simulink model "project4"  (R2020b)
settings: Solver=VariableStepAuto  StartTime=0.0  StopTime=5  RelTol=1e-3
libraries: simulink x1, commutil2 x1
settings Model: Creator=derek  LastModifiedBy=hp

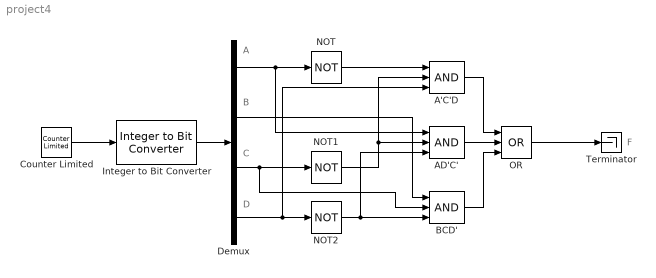
== system project4 ==
  note: A
  note: B
  note: C
  note: D
  note: F
  A'C'D : Logic  Inputs=3  IconShape=distinctive  AllPortsSameDT=off  OutDataTypeStr=boolean
  AD'C' : Logic  Inputs=3  IconShape=distinctive  AllPortsSameDT=off  OutDataTypeStr=boolean
  BCD' : Logic  Inputs=3  IconShape=distinctive  AllPortsSameDT=off  OutDataTypeStr=boolean
  Counter Limited : simulink/Sources/Counter Limited  uplimit=15  tsamp=1
  Demux : Demux
  Integer to Bit Converter : commutil2/Integer to Bit Converter  nbits=4  signedInputValues=Unsigned  bitOrder=MSB first  outDtype=Inherit via internal rule
  NOT : Logic  Operator=NOT  IconShape=distinctive  AllPortsSameDT=off  OutDataTypeStr=boolean
  NOT1 : Logic  Operator=NOT  IconShape=distinctive  AllPortsSameDT=off  OutDataTypeStr=boolean
  NOT2 : Logic  Operator=NOT  IconShape=distinctive  AllPortsSameDT=off  OutDataTypeStr=boolean
  OR : Logic  Operator=OR  Inputs=3  IconShape=distinctive  AllPortsSameDT=off  OutDataTypeStr=boolean
  Terminator : Terminator
  wires:
  Counter Limited/1 -> Integer to Bit Converter/1
  Integer to Bit Converter/1 -> Demux/1
  Demux/1 -> AD'C'/1, NOT/1
  Demux/3 -> BCD'/2, NOT1/1
  Demux/4 -> NOT2/1, A'C'D/3
  NOT/1 -> A'C'D/1
  NOT1/1 -> A'C'D/2, AD'C'/2
  NOT2/1 -> BCD'/3, AD'C'/3
  Demux/2 -> BCD'/1
  A'C'D/1 -> OR/1
  AD'C'/1 -> OR/2
  BCD'/1 -> OR/3
  OR/1 -> Terminator/1
